simulink library "inp"  (R2021b)
settings: Solver=VariableStepAuto  StartTime=0.0  StopTime=10.0  RelTol=1e-3
undefined symbols (not defined in the file): C_TASK_5MS_S, FALSE, KINP_AcoreReadyToSlp_flg_ovrdflg, KINP_AcoreReadyToSlp_flg_ovrdval, KINP_AllowMovThd_OTA_enum_ovrdflg, KINP_AllowMovThd_OTA_enum_ovrdval, KINP_APSAngleTarget_Deg_ovrdflg, KINP_APSAngleTarget_Deg_ovrdval, KINP_APSDecReq_mps2_ovrdflg, KINP_APSDecReq_mps2_ovrdval, KINP_APSDecReqA_flg_ovrdflg, KINP_APSDecReqA_flg_ovrdval, KINP_APSDFLL_cm_ovrdflg, KINP_APSDFLL_cm_ovrdval, KINP_APSDFLR_cm_ovrdflg, KINP_APSDFLR_cm_ovrdval, KINP_APSDRLL_cm_ovrdflg, KINP_APSDRLL_cm_ovrdval, KINP_APSDRLR_cm_ovrdflg, KINP_APSDRLR_cm_ovrdval, KINP_APSExitCondition_enum_ovrdflg, KINP_APSExitCondition_enum_ovrdval, KINP_APSHWVer_enum_ovrdflg, KINP_APSHWVer_enum_ovrdval, KINP_APSProgressPCT_pct_ovrdflg, KINP_APSProgressPCT_pct_ovrdval, KINP_APSPwrReq_enum_ovrdflg, KINP_APSPwrReq_enum_ovrdval, KINP_APSReq_enum_ovrdflg, KINP_APSReq_enum_ovrdval, KINP_APSRQDisplay_enum_ovrdflg, KINP_APSRQDisplay_enum_ovrdval, KINP_APSRqEPASCtrl_flg_ovrdflg, KINP_APSRqEPASCtrl_flg_ovrdval, KINP_APSShiftPosnReq_enum_ovrdval, KINP_APSShiftPosnReq_enum_ovrflg, KINP_APSSpeedCMD_kph_ovrdval, KINP_APSSpeedCMD_kph_ovrflg, KINP_APSStaSystem_enum_ovrdflg, KINP_APSStaSystem_enum_ovrdval, KINP_APSSWVer_enum_ovrdflg, KINP_APSSWVer_enum_ovrdval, KINP_APSVMCReqA_flg_ovrdval, KINP_APSVMCReqA_flg_ovrflg, KINP_APSVRqEPASCtrl_flg_ovrdflg, KINP_APSVRqEPASCtrl_flg_ovrdval, KINP_AuxBattVolmV_mV_ovrdflg, KINP_AuxBattVolmV_mV_ovrdval, KINP_CAASSta_enum_ovrdflg, KINP_CAASSta_enum_ovrdval, KINP_CAASVMCReqA_flg_ovrdval, KINP_CAASVMCReqA_flg_ovrflg, KINP_CAN1BusOff_flg_ovrdflg, KINP_CAN1BusOff_flg_ovrdval, KINP_CAN2BusOff_flg_ovrdflg, KINP_CAN2BusOff_flg_ovrdval, KINP_CAN3BusOff_flg_ovrdflg, KINP_CAN3BusOff_flg_ovrdval, KINP_CAN4BusOff_flg_ovrdflg, KINP_CAN4BusOff_flg_ovrdval ... (+152)
libraries: FVT_lib x1035, hcu_lib x1
(part 4 of 33)

== system inp/INP/CAN1/CreateBus ==
  inp_CanValid_bus : Inport
  inp_Hal_bus : Inport  Port=2
  UnitConverter_{1..13,16,18..27,29,31..32,34..35,41,43..55,58..60,62,64..65,68..73,75,77,80,82,84..85,87,89,92,94,97..100,102..107,109..111,116..117,120,122,124,128,130..134} (89 alike) : DataTypeConversion  OutDataTypeStr=boolean
  UnitConverter_{40,42,66..67,76,81,88,93,96,101,108,118..119,121,123,125,127,129} (18 alike) : DataTypeConversion  OutDataTypeStr=single
  UnitConverter_{14..15,17,28,30,33,36..39,56..57,61,63,74,78..79,83,86,90..91,95,112..115,126} (27 alike) : DataTypeConversion  OutDataTypeStr=uint8
  bus_creator : BusCreator  Inputs=134
  bus_selector : BusSelector  OutputSignals=VINP_CANMsgValidABM1_flg,VINP_CANMsgValidEPB1_flg,VINP_CANMsgValidEPS1_flg,VINP_CANMsgValidESC1_flg,VINP_CANMsgValidESC5_flg,VINP_CANMsgValideBST1_flg
  bus_selector_1 : BusSelector  OutputSignals=VINP_ABM1CSErr_flg,VINP_ABM1RCErr_flg,VINP_ABMPassengerODSSta_flg,VINP_ABMRearPassengerCTRODSSta_flg,VINP_ABMRearPassengerLHODSSta_flg,VINP_ABMRearPassengerRHODSSta_flg,VINP_AirBagFailCmd_flg,VINP_ChecksumABM1_enum,VINP_CrashOutputSts_enum,VINP_DriverSeatBeltCmd_flg,VINP_LifeCountABM1_enum,VINP_PABSwitchCmd_flg,VINP_PsngrSeatBeltCmd_flg,VINP_RCenterSeatBeltCmd_flg,VINP_RDriverSeatBeltCmd_flg,VINP_RPsngrSeatBeltCmd_flg,VINP_TLHPsngrSeatBeltCmd_flg,VINP_TRHPsngrSeatBeltCmd_flg,VINP_EPB1CSErr_flg,VINP_EPB1RCErr_flg,VINP_DOASta_flg,VINP_EPB1RC_enum,VINP_EPBCarWashMode_flg,VINP_EPBErrSta_enum,VINP_EPBExtApplyAvail_flg,VINP_EPBExtReleaseAvail_flg,VINP_EPBSta_enum,VINP_EPS1CSErr_flg,VINP_EPS1RCErr_flg,VINP_DriIntend_enum,VINP_EPSAOIControl_enum,VINP_EPSRC_enum,VINP_EpasFailed_enum,VINP_SASAngle_Deg,VINP_SASCAL_flg,VINP_SASSpeed_degps,VINP_SASSpeedValid_flg,VINP_SASV_flg,VINP_ESC1CSErr_flg,VINP_ESC1RCErr_flg,VINP_ABSActive_flg,VINP_ABSFailed_flg,VINP_ABSWnlmpSta_flg,VINP_AVHActive_flg,VINP_AVHFailed_flg,VINP_AmberWnlmpSta_flg,VINP_BTCSActive_flg,VINP_EBDActive_flg,VINP_EBDFailed_flg,VINP_ESC1CS_enum,VINP_ESC1RC_enum,VINP_ESCActive_flg,VINP_ESCBeepReq_flg,VINP_ESCFailed_flg,VINP_ESCOFFStatus_enum,VINP_ESCOfflmpSta_flg,VINP_ESCWnlmpSta_enum,VINP_ESSActive_flg,VINP_FrPTCSActive_flg,VINP_FrntAxlTrqReqDrv_Nm,VINP_GRADE_Deg,VINP_HBBActive_flg,VINP_HBBFailed_flg,VINP_HDDActive_flg,VINP_HDDFailed_flg,VINP_HSAActive_flg,VINP_HSAFailed_flg,VINP_LFPulseCount_enum,VINP_LFPulseCountV_flg,VINP_LFRawWhlSpeed_kph,VINP_LFRawWhlSpeedV_flg,VINP_LFWhlRotDir_enum,VINP_LRPulseCount_enum,VINP_LRPulseCountV_flg,VINP_LRRawWhlSpeed_kph,VINP_LRRawWhlSpeedV_flg,VINP_LRWhlRotDir_enum,VINP_PBAActive_flg,VINP_PBAFailed_flg,VINP_RFPulseCount_enum,VINP_RFPulseCountV_flg,VINP_RFRawWhlSpeed_kph,VINP_RFRawWhlSpeedV_flg,VINP_RFWhlRotDir_enum,VINP_RRPulseCount_enum,VINP_RRPulseCountV_flg,VINP_RRRawWhlSpeed_kph,VINP_RRRawWhlSpeedV_flg,VINP_RRWhlRotDir_enum,VINP_RearAxlTrqReqDrv_Nm,VINP_RedWnlmpSta_flg,VINP_RrPTCSActive_flg,VINP_TCSActive_flg,VINP_TCSFailed_flg,VINP_VehSpeed_kph,VINP_ESC5CSErr_flg,VINP_ESC5RCErr_flg,VINP_ACCAvail_flg,VINP_AEBAvail_flg,VINP_ActBrkLampSta_flg,VINP_BrkDiscTempSta_flg,VINP_BrkPedalPos_pct,VINP_BrkPedalPosSta_flg,VINP_BrkSwSta_flg,VINP_BrkSwV_flg,VINP_ESC5CS_enum,VINP_ESC5RC_enum,VINP_ESCADASSta_enum,VINP_ESCAPSSta_enum,VINP_ESCStandstill_flg,VINP_FrRBCActive_flg,VINP_FrntAxlTrqReqBrk_Nm,VINP_LatAccel_Gps,VINP_LatAccelV_flg,VINP_LongAccel_Gps,VINP_LongAccelV_flg,VINP_MCPressure_bar,VINP_MCPressureV_flg,VINP_MeterIndVehSpeed_kph,VINP_RDCActive_enum,VINP_RearAxlTrqReqBrk_Nm,VINP_RrRBCActive_flg,VINP_YawRate_degps,VINP_YawRateV_flg,VINP_LowBrakeFluidSta_flg,VINP_eBSTAmberWnlmpSta_flg,VINP_eBSTBeepReq_flg,VINP_eBSTRedWnlmpSta_flg
  BINP_outputs : Outport
  wires:
  inp_CanValid_bus/1 -> [inp_CanValid_bus]
  inp_Hal_bus/1 -> [inp_Hal_bus]
  bus_selector/1 -> UnitConverter_1/1  "<VINP_CANMsgValidABM1_flg>"
  UnitConverter_1/1 -> bus_creator/1  "VINP_CANMsgValidABM1_flg"
  bus_selector/2 -> UnitConverter_2/1  "<VINP_CANMsgValidEPB1_flg>"
  UnitConverter_2/1 -> bus_creator/2  "VINP_CANMsgValidEPB1_flg"
  bus_selector/3 -> UnitConverter_3/1  "<VINP_CANMsgValidEPS1_flg>"
  UnitConverter_3/1 -> bus_creator/3  "VINP_CANMsgValidEPS1_flg"
  bus_selector/4 -> UnitConverter_4/1  "<VINP_CANMsgValidESC1_flg>"
  UnitConverter_4/1 -> bus_creator/4  "VINP_CANMsgValidESC1_flg"
  bus_selector/5 -> UnitConverter_5/1  "<VINP_CANMsgValidESC5_flg>"
  UnitConverter_5/1 -> bus_creator/5  "VINP_CANMsgValidESC5_flg"
  bus_selector/6 -> UnitConverter_6/1  "<VINP_CANMsgValideBST1_flg>"
  UnitConverter_6/1 -> bus_creator/6  "VINP_CANMsgValideBST1_flg"
  bus_selector_1/1 -> UnitConverter_7/1  "<VINP_ABM1CSErr_flg>"
  UnitConverter_7/1 -> bus_creator/7  "VINP_ABM1CSErr_flg"
  bus_selector_1/2 -> UnitConverter_8/1  "<VINP_ABM1RCErr_flg>"
  UnitConverter_8/1 -> bus_creator/8  "VINP_ABM1RCErr_flg"
  bus_selector_1/3 -> UnitConverter_9/1  "<VINP_ABMPassengerODSSta_flg>"
  UnitConverter_9/1 -> bus_creator/9  "VINP_ABMPassengerODSSta_flg"
  bus_selector_1/4 -> UnitConverter_10/1  "<VINP_ABMRearPassengerCTRODSSta_flg>"
  UnitConverter_10/1 -> bus_creator/10  "VINP_ABMRearPassengerCTRODSSta_flg"
  bus_selector_1/5 -> UnitConverter_11/1  "<VINP_ABMRearPassengerLHODSSta_flg>"
  UnitConverter_11/1 -> bus_creator/11  "VINP_ABMRearPassengerLHODSSta_flg"
  bus_selector_1/6 -> UnitConverter_12/1  "<VINP_ABMRearPassengerRHODSSta_flg>"
  UnitConverter_12/1 -> bus_creator/12  "VINP_ABMRearPassengerRHODSSta_flg"
  bus_selector_1/7 -> UnitConverter_13/1  "<VINP_AirBagFailCmd_flg>"
  UnitConverter_13/1 -> bus_creator/13  "VINP_AirBagFailCmd_flg"
  bus_selector_1/8 -> UnitConverter_14/1  "<VINP_ChecksumABM1_enum>"
  UnitConverter_14/1 -> bus_creator/14  "VINP_ChecksumABM1_enum"
  bus_selector_1/9 -> UnitConverter_15/1  "<VINP_CrashOutputSts_enum>"
  UnitConverter_15/1 -> bus_creator/15  "VINP_CrashOutputSts_enum"
  bus_selector_1/10 -> UnitConverter_16/1  "<VINP_DriverSeatBeltCmd_flg>"
  UnitConverter_16/1 -> bus_creator/16  "VINP_DriverSeatBeltCmd_flg"
  bus_selector_1/11 -> UnitConverter_17/1  "<VINP_LifeCountABM1_enum>"
  UnitConverter_17/1 -> bus_creator/17  "VINP_LifeCountABM1_enum"
  bus_selector_1/12 -> UnitConverter_18/1  "<VINP_PABSwitchCmd_flg>"
  UnitConverter_18/1 -> bus_creator/18  "VINP_PABSwitchCmd_flg"
  bus_selector_1/13 -> UnitConverter_19/1  "<VINP_PsngrSeatBeltCmd_flg>"
  UnitConverter_19/1 -> bus_creator/19  "VINP_PsngrSeatBeltCmd_flg"
  bus_selector_1/14 -> UnitConverter_20/1  "<VINP_RCenterSeatBeltCmd_flg>"
  UnitConverter_20/1 -> bus_creator/20  "VINP_RCenterSeatBeltCmd_flg"
  bus_selector_1/15 -> UnitConverter_21/1  "<VINP_RDriverSeatBeltCmd_flg>"
  UnitConverter_21/1 -> bus_creator/21  "VINP_RDriverSeatBeltCmd_flg"
  bus_selector_1/16 -> UnitConverter_22/1  "<VINP_RPsngrSeatBeltCmd_flg>"
  UnitConverter_22/1 -> bus_creator/22  "VINP_RPsngrSeatBeltCmd_flg"
  bus_selector_1/17 -> UnitConverter_23/1  "<VINP_TLHPsngrSeatBeltCmd_flg>"
  UnitConverter_23/1 -> bus_creator/23  "VINP_TLHPsngrSeatBeltCmd_flg"
  bus_selector_1/18 -> UnitConverter_24/1  "<VINP_TRHPsngrSeatBeltCmd_flg>"
  UnitConverter_24/1 -> bus_creator/24  "VINP_TRHPsngrSeatBeltCmd_flg"
  bus_selector_1/19 -> UnitConverter_25/1  "<VINP_EPB1CSErr_flg>"
  UnitConverter_25/1 -> bus_creator/25  "VINP_EPB1CSErr_flg"
  bus_selector_1/20 -> UnitConverter_26/1  "<VINP_EPB1RCErr_flg>"
  UnitConverter_26/1 -> bus_creator/26  "VINP_EPB1RCErr_flg"
  bus_selector_1/21 -> UnitConverter_27/1  "<VINP_DOASta_flg>"
  UnitConverter_27/1 -> bus_creator/27  "VINP_DOASta_flg"
  bus_selector_1/22 -> UnitConverter_28/1  "<VINP_EPB1RC_enum>"
  UnitConverter_28/1 -> bus_creator/28  "VINP_EPB1RC_enum"
  bus_selector_1/23 -> UnitConverter_29/1  "<VINP_EPBCarWashMode_flg>"
  UnitConverter_29/1 -> bus_creator/29  "VINP_EPBCarWashMode_flg"
  bus_selector_1/24 -> UnitConverter_30/1  "<VINP_EPBErrSta_enum>"
  UnitConverter_30/1 -> bus_creator/30  "VINP_EPBErrSta_enum"
  bus_selector_1/25 -> UnitConverter_31/1  "<VINP_EPBExtApplyAvail_flg>"
  UnitConverter_31/1 -> bus_creator/31  "VINP_EPBExtApplyAvail_flg"
  bus_selector_1/26 -> UnitConverter_32/1  "<VINP_EPBExtReleaseAvail_flg>"
  UnitConverter_32/1 -> bus_creator/32  "VINP_EPBExtReleaseAvail_flg"
  bus_selector_1/27 -> UnitConverter_33/1  "<VINP_EPBSta_enum>"
  UnitConverter_33/1 -> bus_creator/33  "VINP_EPBSta_enum"
  bus_selector_1/28 -> UnitConverter_34/1  "<VINP_EPS1CSErr_flg>"
  UnitConverter_34/1 -> bus_creator/34  "VINP_EPS1CSErr_flg"
  bus_selector_1/29 -> UnitConverter_35/1  "<VINP_EPS1RCErr_flg>"
  UnitConverter_35/1 -> bus_creator/35  "VINP_EPS1RCErr_flg"
  bus_selector_1/30 -> UnitConverter_36/1  "<VINP_DriIntend_enum>"
  UnitConverter_36/1 -> bus_creator/36  "VINP_DriIntend_enum"
  bus_selector_1/31 -> UnitConverter_37/1  "<VINP_EPSAOIControl_enum>"
  UnitConverter_37/1 -> bus_creator/37  "VINP_EPSAOIControl_enum"
  bus_selector_1/32 -> UnitConverter_38/1  "<VINP_EPSRC_enum>"
  UnitConverter_38/1 -> bus_creator/38  "VINP_EPSRC_enum"
  bus_selector_1/33 -> UnitConverter_39/1  "<VINP_EpasFailed_enum>"
  UnitConverter_39/1 -> bus_creator/39  "VINP_EpasFailed_enum"
  bus_selector_1/34 -> UnitConverter_40/1  "<VINP_SASAngle_Deg>"
  UnitConverter_40/1 -> bus_creator/40  "VINP_SASAngle_Deg"
  bus_selector_1/35 -> UnitConverter_41/1  "<VINP_SASCAL_flg>"
  UnitConverter_41/1 -> bus_creator/41  "VINP_SASCAL_flg"
  bus_selector_1/36 -> UnitConverter_42/1  "<VINP_SASSpeed_degps>"
  UnitConverter_42/1 -> bus_creator/42  "VINP_SASSpeed_degps"
  bus_selector_1/37 -> UnitConverter_43/1  "<VINP_SASSpeedValid_flg>"
  UnitConverter_43/1 -> bus_creator/43  "VINP_SASSpeedValid_flg"
  bus_selector_1/38 -> UnitConverter_44/1  "<VINP_SASV_flg>"
  UnitConverter_44/1 -> bus_creator/44  "VINP_SASV_flg"
  bus_selector_1/39 -> UnitConverter_45/1  "<VINP_ESC1CSErr_flg>"
  UnitConverter_45/1 -> bus_creator/45  "VINP_ESC1CSErr_flg"
  bus_selector_1/40 -> UnitConverter_46/1  "<VINP_ESC1RCErr_flg>"
  UnitConverter_46/1 -> bus_creator/46  "VINP_ESC1RCErr_flg"
  bus_selector_1/41 -> UnitConverter_47/1  "<VINP_ABSActive_flg>"
  UnitConverter_47/1 -> bus_creator/47  "VINP_ABSActive_flg"
  bus_selector_1/42 -> UnitConverter_48/1  "<VINP_ABSFailed_flg>"
  UnitConverter_48/1 -> bus_creator/48  "VINP_ABSFailed_flg"
  bus_selector_1/43 -> UnitConverter_49/1  "<VINP_ABSWnlmpSta_flg>"
  UnitConverter_49/1 -> bus_creator/49  "VINP_ABSWnlmpSta_flg"
  bus_selector_1/44 -> UnitConverter_50/1  "<VINP_AVHActive_flg>"
  UnitConverter_50/1 -> bus_creator/50  "VINP_AVHActive_flg"
  bus_selector_1/45 -> UnitConverter_51/1  "<VINP_AVHFailed_flg>"
  UnitConverter_51/1 -> bus_creator/51  "VINP_AVHFailed_flg"
  bus_selector_1/46 -> UnitConverter_52/1  "<VINP_AmberWnlmpSta_flg>"
  UnitConverter_52/1 -> bus_creator/52  "VINP_AmberWnlmpSta_flg"
  bus_selector_1/47 -> UnitConverter_53/1  "<VINP_BTCSActive_flg>"
  UnitConverter_53/1 -> bus_creator/53  "VINP_BTCSActive_flg"
  bus_selector_1/48 -> UnitConverter_54/1  "<VINP_EBDActive_flg>"
  UnitConverter_54/1 -> bus_creator/54  "VINP_EBDActive_flg"
  bus_selector_1/49 -> UnitConverter_55/1  "<VINP_EBDFailed_flg>"
  UnitConverter_55/1 -> bus_creator/55  "VINP_EBDFailed_flg"
  bus_selector_1/50 -> UnitConverter_56/1  "<VINP_ESC1CS_enum>"
  UnitConverter_56/1 -> bus_creator/56  "VINP_ESC1CS_enum"
  bus_selector_1/51 -> UnitConverter_57/1  "<VINP_ESC1RC_enum>"
  UnitConverter_57/1 -> bus_creator/57  "VINP_ESC1RC_enum"
  bus_selector_1/52 -> UnitConverter_58/1  "<VINP_ESCActive_flg>"
  UnitConverter_58/1 -> bus_creator/58  "VINP_ESCActive_flg"
  bus_selector_1/53 -> UnitConverter_59/1  "<VINP_ESCBeepReq_flg>"
  UnitConverter_59/1 -> bus_creator/59  "VINP_ESCBeepReq_flg"
  bus_selector_1/54 -> UnitConverter_60/1  "<VINP_ESCFailed_flg>"
  UnitConverter_60/1 -> bus_creator/60  "VINP_ESCFailed_flg"
  bus_selector_1/55 -> UnitConverter_61/1  "<VINP_ESCOFFStatus_enum>"
  UnitConverter_61/1 -> bus_creator/61  "VINP_ESCOFFStatus_enum"
  bus_selector_1/56 -> UnitConverter_62/1  "<VINP_ESCOfflmpSta_flg>"
  UnitConverter_62/1 -> bus_creator/62  "VINP_ESCOfflmpSta_flg"
  bus_selector_1/57 -> UnitConverter_63/1  "<VINP_ESCWnlmpSta_enum>"
  UnitConverter_63/1 -> bus_creator/63  "VINP_ESCWnlmpSta_enum"
  bus_selector_1/58 -> UnitConverter_64/1  "<VINP_ESSActive_flg>"
  UnitConverter_64/1 -> bus_creator/64  "VINP_ESSActive_flg"
  bus_selector_1/59 -> UnitConverter_65/1  "<VINP_FrPTCSActive_flg>"
  UnitConverter_65/1 -> bus_creator/65  "VINP_FrPTCSActive_flg"
  bus_selector_1/60 -> UnitConverter_66/1  "<VINP_FrntAxlTrqReqDrv_Nm>"
  UnitConverter_66/1 -> bus_creator/66  "VINP_FrntAxlTrqReqDrv_Nm"
  bus_selector_1/61 -> UnitConverter_67/1  "<VINP_GRADE_Deg>"
  UnitConverter_67/1 -> bus_creator/67  "VINP_GRADE_Deg"
  bus_selector_1/62 -> UnitConverter_68/1  "<VINP_HBBActive_flg>"
  UnitConverter_68/1 -> bus_creator/68  "VINP_HBBActive_flg"
  bus_selector_1/63 -> UnitConverter_69/1  "<VINP_HBBFailed_flg>"
  UnitConverter_69/1 -> bus_creator/69  "VINP_HBBFailed_flg"
  bus_selector_1/64 -> UnitConverter_70/1  "<VINP_HDDActive_flg>"
  UnitConverter_70/1 -> bus_creator/70  "VINP_HDDActive_flg"
  bus_selector_1/65 -> UnitConverter_71/1  "<VINP_HDDFailed_flg>"
  UnitConverter_71/1 -> bus_creator/71  "VINP_HDDFailed_flg"
  bus_selector_1/66 -> UnitConverter_72/1  "<VINP_HSAActive_flg>"
  UnitConverter_72/1 -> bus_creator/72  "VINP_HSAActive_flg"
  bus_selector_1/67 -> UnitConverter_73/1  "<VINP_HSAFailed_flg>"
  UnitConverter_73/1 -> bus_creator/73  "VINP_HSAFailed_flg"
  bus_selector_1/68 -> UnitConverter_74/1  "<VINP_LFPulseCount_enum>"
  UnitConverter_74/1 -> bus_creator/74  "VINP_LFPulseCount_enum"
  bus_selector_1/69 -> UnitConverter_75/1  "<VINP_LFPulseCountV_flg>"
  UnitConverter_75/1 -> bus_creator/75  "VINP_LFPulseCountV_flg"
  bus_selector_1/70 -> UnitConverter_76/1  "<VINP_LFRawWhlSpeed_kph>"
  UnitConverter_76/1 -> bus_creator/76  "VINP_LFRawWhlSpeed_kph"
  bus_selector_1/71 -> UnitConverter_77/1  "<VINP_LFRawWhlSpeedV_flg>"
  UnitConverter_77/1 -> bus_creator/77  "VINP_LFRawWhlSpeedV_flg"
  bus_selector_1/72 -> UnitConverter_78/1  "<VINP_LFWhlRotDir_enum>"
  UnitConverter_78/1 -> bus_creator/78  "VINP_LFWhlRotDir_enum"
  bus_selector_1/73 -> UnitConverter_79/1  "<VINP_LRPulseCount_enum>"
  UnitConverter_79/1 -> bus_creator/79  "VINP_LRPulseCount_enum"
  bus_selector_1/74 -> UnitConverter_80/1  "<VINP_LRPulseCountV_flg>"
  UnitConverter_80/1 -> bus_creator/80  "VINP_LRPulseCountV_flg"
  bus_selector_1/75 -> UnitConverter_81/1  "<VINP_LRRawWhlSpeed_kph>"
  UnitConverter_81/1 -> bus_creator/81  "VINP_LRRawWhlSpeed_kph"
  bus_selector_1/76 -> UnitConverter_82/1  "<VINP_LRRawWhlSpeedV_flg>"
  UnitConverter_82/1 -> bus_creator/82  "VINP_LRRawWhlSpeedV_flg"
  bus_selector_1/77 -> UnitConverter_83/1  "<VINP_LRWhlRotDir_enum>"
  UnitConverter_83/1 -> bus_creator/83  "VINP_LRWhlRotDir_enum"
  bus_selector_1/78 -> UnitConverter_84/1  "<VINP_PBAActive_flg>"
  UnitConverter_84/1 -> bus_creator/84  "VINP_PBAActive_flg"
  bus_selector_1/79 -> UnitConverter_85/1  "<VINP_PBAFailed_flg>"
  UnitConverter_85/1 -> bus_creator/85  "VINP_PBAFailed_flg"
  bus_selector_1/80 -> UnitConverter_86/1  "<VINP_RFPulseCount_enum>"
  UnitConverter_86/1 -> bus_creator/86  "VINP_RFPulseCount_enum"
  bus_selector_1/81 -> UnitConverter_87/1  "<VINP_RFPulseCountV_flg>"
  UnitConverter_87/1 -> bus_creator/87  "VINP_RFPulseCountV_flg"
  bus_selector_1/82 -> UnitConverter_88/1  "<VINP_RFRawWhlSpeed_kph>"
  UnitConverter_88/1 -> bus_creator/88  "VINP_RFRawWhlSpeed_kph"
  bus_selector_1/83 -> UnitConverter_89/1  "<VINP_RFRawWhlSpeedV_flg>"
  UnitConverter_89/1 -> bus_creator/89  "VINP_RFRawWhlSpeedV_flg"
  bus_selector_1/84 -> UnitConverter_90/1  "<VINP_RFWhlRotDir_enum>"
  UnitConverter_90/1 -> bus_creator/90  "VINP_RFWhlRotDir_enum"
  bus_selector_1/85 -> UnitConverter_91/1  "<VINP_RRPulseCount_enum>"
  UnitConverter_91/1 -> bus_creator/91  "VINP_RRPulseCount_enum"
  bus_selector_1/86 -> UnitConverter_92/1  "<VINP_RRPulseCountV_flg>"
  UnitConverter_92/1 -> bus_creator/92  "VINP_RRPulseCountV_flg"
  bus_selector_1/87 -> UnitConverter_93/1  "<VINP_RRRawWhlSpeed_kph>"
  UnitConverter_93/1 -> bus_creator/93  "VINP_RRRawWhlSpeed_kph"
  bus_selector_1/88 -> UnitConverter_94/1  "<VINP_RRRawWhlSpeedV_flg>"
  UnitConverter_94/1 -> bus_creator/94  "VINP_RRRawWhlSpeedV_flg"
  bus_selector_1/89 -> UnitConverter_95/1  "<VINP_RRWhlRotDir_enum>"
  UnitConverter_95/1 -> bus_creator/95  "VINP_RRWhlRotDir_enum"
  bus_selector_1/90 -> UnitConverter_96/1  "<VINP_RearAxlTrqReqDrv_Nm>"
  UnitConverter_96/1 -> bus_creator/96  "VINP_RearAxlTrqReqDrv_Nm"
  bus_selector_1/91 -> UnitConverter_97/1  "<VINP_RedWnlmpSta_flg>"
  UnitConverter_97/1 -> bus_creator/97  "VINP_RedWnlmpSta_flg"
  bus_selector_1/92 -> UnitConverter_98/1  "<VINP_RrPTCSActive_flg>"
  UnitConverter_98/1 -> bus_creator/98  "VINP_RrPTCSActive_flg"
  bus_selector_1/93 -> UnitConverter_99/1  "<VINP_TCSActive_flg>"
  UnitConverter_99/1 -> bus_creator/99  "VINP_TCSActive_flg"
  bus_selector_1/94 -> UnitConverter_100/1  "<VINP_TCSFailed_flg>"
  UnitConverter_100/1 -> bus_creator/100  "VINP_TCSFailed_flg"
  bus_selector_1/95 -> UnitConverter_101/1  "<VINP_VehSpeed_kph>"
  UnitConverter_101/1 -> bus_creator/101  "VINP_VehSpeed_kph"
  bus_selector_1/96 -> UnitConverter_102/1  "<VINP_ESC5CSErr_flg>"
  UnitConverter_102/1 -> bus_creator/102  "VINP_ESC5CSErr_flg"
  bus_selector_1/97 -> UnitConverter_103/1  "<VINP_ESC5RCErr_flg>"
  UnitConverter_103/1 -> bus_creator/103  "VINP_ESC5RCErr_flg"
  bus_selector_1/98 -> UnitConverter_104/1  "<VINP_ACCAvail_flg>"
  UnitConverter_104/1 -> bus_creator/104  "VINP_ACCAvail_flg"
  bus_selector_1/99 -> UnitConverter_105/1  "<VINP_AEBAvail_flg>"
  UnitConverter_105/1 -> bus_creator/105  "VINP_AEBAvail_flg"
  bus_selector_1/100 -> UnitConverter_106/1  "<VINP_ActBrkLampSta_flg>"
  UnitConverter_106/1 -> bus_creator/106  "VINP_ActBrkLampSta_flg"
  bus_selector_1/101 -> UnitConverter_107/1  "<VINP_BrkDiscTempSta_flg>"
  UnitConverter_107/1 -> bus_creator/107  "VINP_BrkDiscTempSta_flg"
  bus_selector_1/102 -> UnitConverter_108/1  "<VINP_BrkPedalPos_pct>"
  UnitConverter_108/1 -> bus_creator/108  "VINP_BrkPedalPos_pct"
  bus_selector_1/103 -> UnitConverter_109/1  "<VINP_BrkPedalPosSta_flg>"
  UnitConverter_109/1 -> bus_creator/109  "VINP_BrkPedalPosSta_flg"
  bus_selector_1/104 -> UnitConverter_110/1  "<VINP_BrkSwSta_flg>"
  UnitConverter_110/1 -> bus_creator/110  "VINP_BrkSwSta_flg"
  bus_selector_1/105 -> UnitConverter_111/1  "<VINP_BrkSwV_flg>"
  UnitConverter_111/1 -> bus_creator/111  "VINP_BrkSwV_flg"
  bus_selector_1/106 -> UnitConverter_112/1  "<VINP_ESC5CS_enum>"
  UnitConverter_112/1 -> bus_creator/112  "VINP_ESC5CS_enum"
  bus_selector_1/107 -> UnitConverter_113/1  "<VINP_ESC5RC_enum>"
  UnitConverter_113/1 -> bus_creator/113  "VINP_ESC5RC_enum"
  bus_selector_1/108 -> UnitConverter_114/1  "<VINP_ESCADASSta_enum>"
  UnitConverter_114/1 -> bus_creator/114  "VINP_ESCADASSta_enum"
  bus_selector_1/109 -> UnitConverter_115/1  "<VINP_ESCAPSSta_enum>"
  UnitConverter_115/1 -> bus_creator/115  "VINP_ESCAPSSta_enum"
  bus_selector_1/110 -> UnitConverter_116/1  "<VINP_ESCStandstill_flg>"
  UnitConverter_116/1 -> bus_creator/116  "VINP_ESCStandstill_flg"
  bus_selector_1/111 -> UnitConverter_117/1  "<VINP_FrRBCActive_flg>"
  UnitConverter_117/1 -> bus_creator/117  "VINP_FrRBCActive_flg"
  bus_selector_1/112 -> UnitConverter_118/1  "<VINP_FrntAxlTrqReqBrk_Nm>"
  UnitConverter_118/1 -> bus_creator/118  "VINP_FrntAxlTrqReqBrk_Nm"
  bus_selector_1/113 -> UnitConverter_119/1  "<VINP_LatAccel_Gps>"
  UnitConverter_119/1 -> bus_creator/119  "VINP_LatAccel_Gps"
  bus_selector_1/114 -> UnitConverter_120/1  "<VINP_LatAccelV_flg>"
  UnitConverter_120/1 -> bus_creator/120  "VINP_LatAccelV_flg"
  bus_selector_1/115 -> UnitConverter_121/1  "<VINP_LongAccel_Gps>"
  UnitConverter_121/1 -> bus_creator/121  "VINP_LongAccel_Gps"
  bus_selector_1/116 -> UnitConverter_122/1  "<VINP_LongAccelV_flg>"
  UnitConverter_122/1 -> bus_creator/122  "VINP_LongAccelV_flg"
  bus_selector_1/117 -> UnitConverter_123/1  "<VINP_MCPressure_bar>"
  UnitConverter_123/1 -> bus_creator/123  "VINP_MCPressure_bar"
  bus_selector_1/118 -> UnitConverter_124/1  "<VINP_MCPressureV_flg>"
  UnitConverter_124/1 -> bus_creator/124  "VINP_MCPressureV_flg"
  bus_selector_1/119 -> UnitConverter_125/1  "<VINP_MeterIndVehSpeed_kph>"
  UnitConverter_125/1 -> bus_creator/125  "VINP_MeterIndVehSpeed_kph"
  bus_selector_1/120 -> UnitConverter_126/1  "<VINP_RDCActive_enum>"
  UnitConverter_126/1 -> bus_creator/126  "VINP_RDCActive_enum"
  bus_selector_1/121 -> UnitConverter_127/1  "<VINP_RearAxlTrqReqBrk_Nm>"
  UnitConverter_127/1 -> bus_creator/127  "VINP_RearAxlTrqReqBrk_Nm"
  bus_selector_1/122 -> UnitConverter_128/1  "<VINP_RrRBCActive_flg>"
  UnitConverter_128/1 -> bus_creator/128  "VINP_RrRBCActive_flg"
  bus_selector_1/123 -> UnitConverter_129/1  "<VINP_YawRate_degps>"
  UnitConverter_129/1 -> bus_creator/129  "VINP_YawRate_degps"
  bus_selector_1/124 -> UnitConverter_130/1  "<VINP_YawRateV_flg>"
  UnitConverter_130/1 -> bus_creator/130  "VINP_YawRateV_flg"
  bus_selector_1/125 -> UnitConverter_131/1  "<VINP_LowBrakeFluidSta_flg>"
  UnitConverter_131/1 -> bus_creator/131  "VINP_LowBrakeFluidSta_flg"
  bus_selector_1/126 -> UnitConverter_132/1  "<VINP_eBSTAmberWnlmpSta_flg>"
  UnitConverter_132/1 -> bus_creator/132  "VINP_eBSTAmberWnlmpSta_flg"
  bus_selector_1/127 -> UnitConverter_133/1  "<VINP_eBSTBeepReq_flg>"
  UnitConverter_133/1 -> bus_creator/133  "VINP_eBSTBeepReq_flg"
  bus_selector_1/128 -> UnitConverter_134/1  "<VINP_eBSTRedWnlmpSta_flg>"
  UnitConverter_134/1 -> bus_creator/134  "VINP_eBSTRedWnlmpSta_flg"
  [inp_CanValid_bus] -> bus_selector/1
  [inp_Hal_bus] -> bus_selector_1/1
  bus_creator/1 -> BINP_outputs/1

== system inp/INP/CAN1/SignalCheck ==
  inp_CanValid_bus : Inport
  TASK_TIME_S : Inport  Port=2
  BHAL_outputs : Inport  Port=3
  ABM1 : Subsystem
  EPB1 : Subsystem
  EPS1 : Subsystem
  ESC1 : Subsystem
  ESC5 : Subsystem
  bus_creator : BusCreator  Inputs=128
  eBST1 : Subsystem
  inp_Hal_bus : Outport
  wires:
  inp_CanValid_bus/1 -> [inp_CanValid_bus]
  TASK_TIME_S/1 -> [TASK_TIME_S]
  BHAL_outputs/1 -> [BHAL_outputs]
  [BHAL_outputs] -> ABM1/1(BHAL_outputs)
  [inp_CanValid_bus] -> ABM1/2(inp_CanValid_bus)
  ABM1/1(VINP_ABM1CSErr_flg) -> [VINP_ABM1CSErr_flg]
  ABM1/2(VINP_ABM1RCErr_flg) -> [VINP_ABM1RCErr_flg]
  ABM1/3(VINP_ABMPassengerODSSta_flg) -> [VINP_ABMPassengerODSSta_flg]
  ABM1/4(VINP_ABMRearPassengerCTRODSSta_flg) -> [VINP_ABMRearPassengerCTRODSSta_flg]
  ABM1/5(VINP_ABMRearPassengerLHODSSta_flg) -> [VINP_ABMRearPassengerLHODSSta_flg]
  ABM1/6(VINP_ABMRearPassengerRHODSSta_flg) -> [VINP_ABMRearPassengerRHODSSta_flg]
  ABM1/7(VINP_AirBagFailCmd_flg) -> [VINP_AirBagFailCmd_flg]
  ABM1/8(VINP_ChecksumABM1_enum) -> [VINP_ChecksumABM1_enum]
  ABM1/9(VINP_CrashOutputSts_enum) -> [VINP_CrashOutputSts_enum]
  ABM1/10(VINP_DriverSeatBeltCmd_flg) -> [VINP_DriverSeatBeltCmd_flg]
  ABM1/11(VINP_LifeCountABM1_enum) -> [VINP_LifeCountABM1_enum]
  ABM1/12(VINP_PABSwitchCmd_flg) -> [VINP_PABSwitchCmd_flg]
  ABM1/13(VINP_PsngrSeatBeltCmd_flg) -> [VINP_PsngrSeatBeltCmd_flg]
  ABM1/14(VINP_RCenterSeatBeltCmd_flg) -> [VINP_RCenterSeatBeltCmd_flg]
  ABM1/15(VINP_RDriverSeatBeltCmd_flg) -> [VINP_RDriverSeatBeltCmd_flg]
  ABM1/16(VINP_RPsngrSeatBeltCmd_flg) -> [VINP_RPsngrSeatBeltCmd_flg]
  ABM1/17(VINP_TLHPsngrSeatBeltCmd_flg) -> [VINP_TLHPsngrSeatBeltCmd_flg]
  ABM1/18(VINP_TRHPsngrSeatBeltCmd_flg) -> [VINP_TRHPsngrSeatBeltCmd_flg]
  [BHAL_outputs] -> EPB1/1(BHAL_outputs)
  [inp_CanValid_bus] -> EPB1/2(inp_CanValid_bus)
  EPB1/1(VINP_EPB1CSErr_flg) -> [VINP_EPB1CSErr_flg]
  EPB1/2(VINP_EPB1RCErr_flg) -> [VINP_EPB1RCErr_flg]
  EPB1/3(VINP_DOASta_flg) -> [VINP_DOASta_flg]
  EPB1/4(VINP_EPB1RC_enum) -> [VINP_EPB1RC_enum]
  EPB1/5(VINP_EPBCarWashMode_flg) -> [VINP_EPBCarWashMode_flg]
  EPB1/6(VINP_EPBErrSta_enum) -> [VINP_EPBErrSta_enum]
  EPB1/7(VINP_EPBExtApplyAvail_flg) -> [VINP_EPBExtApplyAvail_flg]
  EPB1/8(VINP_EPBExtReleaseAvail_flg) -> [VINP_EPBExtReleaseAvail_flg]
  EPB1/9(VINP_EPBSta_enum) -> [VINP_EPBSta_enum]
  [BHAL_outputs] -> EPS1/1(BHAL_outputs)
  [inp_CanValid_bus] -> EPS1/2(inp_CanValid_bus)
  EPS1/1(VINP_EPS1CSErr_flg) -> [VINP_EPS1CSErr_flg]
  EPS1/2(VINP_EPS1RCErr_flg) -> [VINP_EPS1RCErr_flg]
  EPS1/3(VINP_DriIntend_enum) -> [VINP_DriIntend_enum]
  EPS1/4(VINP_EPSAOIControl_enum) -> [VINP_EPSAOIControl_enum]
  EPS1/5(VINP_EPSRC_enum) -> [VINP_EPSRC_enum]
  EPS1/6(VINP_EpasFailed_enum) -> [VINP_EpasFailed_enum]
  EPS1/7(VINP_SASAngle_Deg) -> [VINP_SASAngle_Deg]
  EPS1/8(VINP_SASCAL_flg) -> [VINP_SASCAL_flg]
  EPS1/9(VINP_SASSpeed_degps) -> [VINP_SASSpeed_degps]
  EPS1/10(VINP_SASSpeedValid_flg) -> [VINP_SASSpeedValid_flg]
  EPS1/11(VINP_SASV_flg) -> [VINP_SASV_flg]
  [BHAL_outputs] -> ESC1/1(BHAL_outputs)
  [inp_CanValid_bus] -> ESC1/2(inp_CanValid_bus)
  ESC1/1(VINP_ESC1CSErr_flg) -> [VINP_ESC1CSErr_flg]
  ESC1/2(VINP_ESC1RCErr_flg) -> [VINP_ESC1RCErr_flg]
  ESC1/3(VINP_ABSActive_flg) -> [VINP_ABSActive_flg]
  ESC1/4(VINP_ABSFailed_flg) -> [VINP_ABSFailed_flg]
  ESC1/5(VINP_ABSWnlmpSta_flg) -> [VINP_ABSWnlmpSta_flg]
  ESC1/6(VINP_AVHActive_flg) -> [VINP_AVHActive_flg]
  ESC1/7(VINP_AVHFailed_flg) -> [VINP_AVHFailed_flg]
  ESC1/8(VINP_AmberWnlmpSta_flg) -> [VINP_AmberWnlmpSta_flg]
  ESC1/9(VINP_BTCSActive_flg) -> [VINP_BTCSActive_flg]
  ESC1/10(VINP_EBDActive_flg) -> [VINP_EBDActive_flg]
  ESC1/11(VINP_EBDFailed_flg) -> [VINP_EBDFailed_flg]
  ESC1/12(VINP_ESC1CS_enum) -> [VINP_ESC1CS_enum]
  ESC1/13(VINP_ESC1RC_enum) -> [VINP_ESC1RC_enum]
  ESC1/14(VINP_ESCActive_flg) -> [VINP_ESCActive_flg]
  ESC1/15(VINP_ESCBeepReq_flg) -> [VINP_ESCBeepReq_flg]
  ESC1/16(VINP_ESCFailed_flg) -> [VINP_ESCFailed_flg]
  ESC1/17(VINP_ESCOFFStatus_enum) -> [VINP_ESCOFFStatus_enum]
  ESC1/18(VINP_ESCOfflmpSta_flg) -> [VINP_ESCOfflmpSta_flg]
  ESC1/19(VINP_ESCWnlmpSta_enum) -> [VINP_ESCWnlmpSta_enum]
  ESC1/20(VINP_ESSActive_flg) -> [VINP_ESSActive_flg]
  ESC1/21(VINP_FrPTCSActive_flg) -> [VINP_FrPTCSActive_flg]
  ESC1/22(VINP_FrntAxlTrqReqDrv_Nm) -> [VINP_FrntAxlTrqReqDrv_Nm]
  ESC1/23(VINP_GRADE_Deg) -> [VINP_GRADE_Deg]
  ESC1/24(VINP_HBBActive_flg) -> [VINP_HBBActive_flg]
  ESC1/25(VINP_HBBFailed_flg) -> [VINP_HBBFailed_flg]
  ESC1/26(VINP_HDDActive_flg) -> [VINP_HDDActive_flg]
  ESC1/27(VINP_HDDFailed_flg) -> [VINP_HDDFailed_flg]
  ESC1/28(VINP_HSAActive_flg) -> [VINP_HSAActive_flg]
  ESC1/29(VINP_HSAFailed_flg) -> [VINP_HSAFailed_flg]
  ESC1/30(VINP_LFPulseCount_enum) -> [VINP_LFPulseCount_enum]
  ESC1/31(VINP_LFPulseCountV_flg) -> [VINP_LFPulseCountV_flg]
  ESC1/32(VINP_LFRawWhlSpeed_kph) -> [VINP_LFRawWhlSpeed_kph]
  ESC1/33(VINP_LFRawWhlSpeedV_flg) -> [VINP_LFRawWhlSpeedV_flg]
  ESC1/34(VINP_LFWhlRotDir_enum) -> [VINP_LFWhlRotDir_enum]
  ESC1/35(VINP_LRPulseCount_enum) -> [VINP_LRPulseCount_enum]
  ESC1/36(VINP_LRPulseCountV_flg) -> [VINP_LRPulseCountV_flg]
  ESC1/37(VINP_LRRawWhlSpeed_kph) -> [VINP_LRRawWhlSpeed_kph]
  ESC1/38(VINP_LRRawWhlSpeedV_flg) -> [VINP_LRRawWhlSpeedV_flg]
  ESC1/39(VINP_LRWhlRotDir_enum) -> [VINP_LRWhlRotDir_enum]
  ESC1/40(VINP_PBAActive_flg) -> [VINP_PBAActive_flg]
  ESC1/41(VINP_PBAFailed_flg) -> [VINP_PBAFailed_flg]
  ESC1/42(VINP_RFPulseCount_enum) -> [VINP_RFPulseCount_enum]
  ESC1/43(VINP_RFPulseCountV_flg) -> [VINP_RFPulseCountV_flg]
  ESC1/44(VINP_RFRawWhlSpeed_kph) -> [VINP_RFRawWhlSpeed_kph]
  ESC1/45(VINP_RFRawWhlSpeedV_flg) -> [VINP_RFRawWhlSpeedV_flg]
  ESC1/46(VINP_RFWhlRotDir_enum) -> [VINP_RFWhlRotDir_enum]
  ESC1/47(VINP_RRPulseCount_enum) -> [VINP_RRPulseCount_enum]
  ESC1/48(VINP_RRPulseCountV_flg) -> [VINP_RRPulseCountV_flg]
  ESC1/49(VINP_RRRawWhlSpeed_kph) -> [VINP_RRRawWhlSpeed_kph]
  ESC1/50(VINP_RRRawWhlSpeedV_flg) -> [VINP_RRRawWhlSpeedV_flg]
  ESC1/51(VINP_RRWhlRotDir_enum) -> [VINP_RRWhlRotDir_enum]
  ESC1/52(VINP_RearAxlTrqReqDrv_Nm) -> [VINP_RearAxlTrqReqDrv_Nm]
  ESC1/53(VINP_RedWnlmpSta_flg) -> [VINP_RedWnlmpSta_flg]
  ESC1/54(VINP_RrPTCSActive_flg) -> [VINP_RrPTCSActive_flg]
  ESC1/55(VINP_TCSActive_flg) -> [VINP_TCSActive_flg]
  ESC1/56(VINP_TCSFailed_flg) -> [VINP_TCSFailed_flg]
  ESC1/57(VINP_VehSpeed_kph) -> [VINP_VehSpeed_kph]
  [BHAL_outputs] -> ESC5/1(BHAL_outputs)
  [inp_CanValid_bus] -> ESC5/2(inp_CanValid_bus)
  ESC5/1(VINP_ESC5CSErr_flg) -> [VINP_ESC5CSErr_flg]
  ESC5/2(VINP_ESC5RCErr_flg) -> [VINP_ESC5RCErr_flg]
  ESC5/3(VINP_ACCAvail_flg) -> [VINP_ACCAvail_flg]
  ESC5/4(VINP_AEBAvail_flg) -> [VINP_AEBAvail_flg]
  ESC5/5(VINP_ActBrkLampSta_flg) -> [VINP_ActBrkLampSta_flg]
  ESC5/6(VINP_BrkDiscTempSta_flg) -> [VINP_BrkDiscTempSta_flg]
  ESC5/7(VINP_BrkPedalPos_pct) -> [VINP_BrkPedalPos_pct]
  ESC5/8(VINP_BrkPedalPosSta_flg) -> [VINP_BrkPedalPosSta_flg]
  ESC5/9(VINP_BrkSwSta_flg) -> [VINP_BrkSwSta_flg]
  ESC5/10(VINP_BrkSwV_flg) -> [VINP_BrkSwV_flg]
  ESC5/11(VINP_ESC5CS_enum) -> [VINP_ESC5CS_enum]
  ESC5/12(VINP_ESC5RC_enum) -> [VINP_ESC5RC_enum]
  ESC5/13(VINP_ESCADASSta_enum) -> [VINP_ESCADASSta_enum]
  ESC5/14(VINP_ESCAPSSta_enum) -> [VINP_ESCAPSSta_enum]
  ESC5/15(VINP_ESCStandstill_flg) -> [VINP_ESCStandstill_flg]
  ESC5/16(VINP_FrRBCActive_flg) -> [VINP_FrRBCActive_flg]
  ESC5/17(VINP_FrntAxlTrqReqBrk_Nm) -> [VINP_FrntAxlTrqReqBrk_Nm]
  ESC5/18(VINP_LatAccel_Gps) -> [VINP_LatAccel_Gps]
  ESC5/19(VINP_LatAccelV_flg) -> [VINP_LatAccelV_flg]
  ESC5/20(VINP_LongAccel_Gps) -> [VINP_LongAccel_Gps]
  ESC5/21(VINP_LongAccelV_flg) -> [VINP_LongAccelV_flg]
  ESC5/22(VINP_MCPressure_bar) -> [VINP_MCPressure_bar]
  ESC5/23(VINP_MCPressureV_flg) -> [VINP_MCPressureV_flg]
  ESC5/24(VINP_MeterIndVehSpeed_kph) -> [VINP_MeterIndVehSpeed_kph]
  ESC5/25(VINP_RDCActive_enum) -> [VINP_RDCActive_enum]
  ESC5/26(VINP_RearAxlTrqReqBrk_Nm) -> [VINP_RearAxlTrqReqBrk_Nm]
  ESC5/27(VINP_RrRBCActive_flg) -> [VINP_RrRBCActive_flg]
  ESC5/28(VINP_YawRate_degps) -> [VINP_YawRate_degps]
  ESC5/29(VINP_YawRateV_flg) -> [VINP_YawRateV_flg]
  [BHAL_outputs] -> eBST1/1(BHAL_outputs)
  [inp_CanValid_bus] -> eBST1/2(inp_CanValid_bus)
  eBST1/1(VINP_LowBrakeFluidSta_flg) -> [VINP_LowBrakeFluidSta_flg]
  eBST1/2(VINP_eBSTAmberWnlmpSta_flg) -> [VINP_eBSTAmberWnlmpSta_flg]
  eBST1/3(VINP_eBSTBeepReq_flg) -> [VINP_eBSTBeepReq_flg]
  eBST1/4(VINP_eBSTRedWnlmpSta_flg) -> [VINP_eBSTRedWnlmpSta_flg]
  bus_creator/1 -> inp_Hal_bus/1
  [VINP_ABM1CSErr_flg] -> bus_creator/1
  [VINP_ABM1RCErr_flg] -> bus_creator/2
  [VINP_ABMPassengerODSSta_flg] -> bus_creator/3
  [VINP_ABMRearPassengerCTRODSSta_flg] -> bus_creator/4
  [VINP_ABMRearPassengerLHODSSta_flg] -> bus_creator/5
  [VINP_ABMRearPassengerRHODSSta_flg] -> bus_creator/6
  [VINP_AirBagFailCmd_flg] -> bus_creator/7
  [VINP_ChecksumABM1_enum] -> bus_creator/8
  [VINP_CrashOutputSts_enum] -> bus_creator/9
  [VINP_DriverSeatBeltCmd_flg] -> bus_creator/10
  [VINP_LifeCountABM1_enum] -> bus_creator/11
  [VINP_PABSwitchCmd_flg] -> bus_creator/12
  [VINP_PsngrSeatBeltCmd_flg] -> bus_creator/13
  [VINP_RCenterSeatBeltCmd_flg] -> bus_creator/14
  [VINP_RDriverSeatBeltCmd_flg] -> bus_creator/15
  [VINP_RPsngrSeatBeltCmd_flg] -> bus_creator/16
  [VINP_TLHPsngrSeatBeltCmd_flg] -> bus_creator/17
  [VINP_TRHPsngrSeatBeltCmd_flg] -> bus_creator/18
  [VINP_EPB1CSErr_flg] -> bus_creator/19
  [VINP_EPB1RCErr_flg] -> bus_creator/20
  [VINP_DOASta_flg] -> bus_creator/21
  [VINP_EPB1RC_enum] -> bus_creator/22
  [VINP_EPBCarWashMode_flg] -> bus_creator/23
  [VINP_EPBErrSta_enum] -> bus_creator/24
  [VINP_EPBExtApplyAvail_flg] -> bus_creator/25
  [VINP_EPBExtReleaseAvail_flg] -> bus_creator/26
  [VINP_EPBSta_enum] -> bus_creator/27
  [VINP_EPS1CSErr_flg] -> bus_creator/28
  [VINP_EPS1RCErr_flg] -> bus_creator/29
  [VINP_DriIntend_enum] -> bus_creator/30
  [VINP_EPSAOIControl_enum] -> bus_creator/31
  [VINP_EPSRC_enum] -> bus_creator/32
  [VINP_EpasFailed_enum] -> bus_creator/33
  [VINP_SASAngle_Deg] -> bus_creator/34
  [VINP_SASCAL_flg] -> bus_creator/35
  [VINP_SASSpeed_degps] -> bus_creator/36
  [VINP_SASSpeedValid_flg] -> bus_creator/37
  [VINP_SASV_flg] -> bus_creator/38
  [VINP_ESC1CSErr_flg] -> bus_creator/39
  [VINP_ESC1RCErr_flg] -> bus_creator/40
  [VINP_ABSActive_flg] -> bus_creator/41
  [VINP_ABSFailed_flg] -> bus_creator/42
  [VINP_ABSWnlmpSta_flg] -> bus_creator/43
  [VINP_AVHActive_flg] -> bus_creator/44
  [VINP_AVHFailed_flg] -> bus_creator/45
  [VINP_AmberWnlmpSta_flg] -> bus_creator/46
  [VINP_BTCSActive_flg] -> bus_creator/47
  [VINP_EBDActive_flg] -> bus_creator/48
  [VINP_EBDFailed_flg] -> bus_creator/49
  [VINP_ESC1CS_enum] -> bus_creator/50
  [VINP_ESC1RC_enum] -> bus_creator/51
  [VINP_ESCActive_flg] -> bus_creator/52
  [VINP_ESCBeepReq_flg] -> bus_creator/53
  [VINP_ESCFailed_flg] -> bus_creator/54
  [VINP_ESCOFFStatus_enum] -> bus_creator/55
  [VINP_ESCOfflmpSta_flg] -> bus_creator/56
  [VINP_ESCWnlmpSta_enum] -> bus_creator/57
  [VINP_ESSActive_flg] -> bus_creator/58
  [VINP_FrPTCSActive_flg] -> bus_creator/59
  [VINP_FrntAxlTrqReqDrv_Nm] -> bus_creator/60
  [VINP_GRADE_Deg] -> bus_creator/61
  [VINP_HBBActive_flg] -> bus_creator/62
  [VINP_HBBFailed_flg] -> bus_creator/63
  [VINP_HDDActive_flg] -> bus_creator/64
  [VINP_HDDFailed_flg] -> bus_creator/65
  [VINP_HSAActive_flg] -> bus_creator/66
  [VINP_HSAFailed_flg] -> bus_creator/67
  [VINP_LFPulseCount_enum] -> bus_creator/68
  [VINP_LFPulseCountV_flg] -> bus_creator/69
  [VINP_LFRawWhlSpeed_kph] -> bus_creator/70
  [VINP_LFRawWhlSpeedV_flg] -> bus_creator/71
  [VINP_LFWhlRotDir_enum] -> bus_creator/72
  [VINP_LRPulseCount_enum] -> bus_creator/73
  [VINP_LRPulseCountV_flg] -> bus_creator/74
  [VINP_LRRawWhlSpeed_kph] -> bus_creator/75
  [VINP_LRRawWhlSpeedV_flg] -> bus_creator/76
  [VINP_LRWhlRotDir_enum] -> bus_creator/77
  [VINP_PBAActive_flg] -> bus_creator/78
  [VINP_PBAFailed_flg] -> bus_creator/79
  [VINP_RFPulseCount_enum] -> bus_creator/80
  [VINP_RFPulseCountV_flg] -> bus_creator/81
  [VINP_RFRawWhlSpeed_kph] -> bus_creator/82
  [VINP_RFRawWhlSpeedV_flg] -> bus_creator/83
  [VINP_RFWhlRotDir_enum] -> bus_creator/84
  [VINP_RRPulseCount_enum] -> bus_creator/85
  [VINP_RRPulseCountV_flg] -> bus_creator/86
  [VINP_RRRawWhlSpeed_kph] -> bus_creator/87
  [VINP_RRRawWhlSpeedV_flg] -> bus_creator/88
  [VINP_RRWhlRotDir_enum] -> bus_creator/89
  [VINP_RearAxlTrqReqDrv_Nm] -> bus_creator/90
  [VINP_RedWnlmpSta_flg] -> bus_creator/91
  [VINP_RrPTCSActive_flg] -> bus_creator/92
  [VINP_TCSActive_flg] -> bus_creator/93
  [VINP_TCSFailed_flg] -> bus_creator/94
  [VINP_VehSpeed_kph] -> bus_creator/95
  [VINP_ESC5CSErr_flg] -> bus_creator/96
  [VINP_ESC5RCErr_flg] -> bus_creator/97
  [VINP_ACCAvail_flg] -> bus_creator/98
  [VINP_AEBAvail_flg] -> bus_creator/99
  [VINP_ActBrkLampSta_flg] -> bus_creator/100
  [VINP_BrkDiscTempSta_flg] -> bus_creator/101
  [VINP_BrkPedalPos_pct] -> bus_creator/102
  [VINP_BrkPedalPosSta_flg] -> bus_creator/103
  [VINP_BrkSwSta_flg] -> bus_creator/104
  [VINP_BrkSwV_flg] -> bus_creator/105
  [VINP_ESC5CS_enum] -> bus_creator/106
  [VINP_ESC5RC_enum] -> bus_creator/107
  [VINP_ESCADASSta_enum] -> bus_creator/108
  [VINP_ESCAPSSta_enum] -> bus_creator/109
  [VINP_ESCStandstill_flg] -> bus_creator/110
  [VINP_FrRBCActive_flg] -> bus_creator/111
  [VINP_FrntAxlTrqReqBrk_Nm] -> bus_creator/112
  [VINP_LatAccel_Gps] -> bus_creator/113
  [VINP_LatAccelV_flg] -> bus_creator/114
  [VINP_LongAccel_Gps] -> bus_creator/115
  [VINP_LongAccelV_flg] -> bus_creator/116
  [VINP_MCPressure_bar] -> bus_creator/117
  [VINP_MCPressureV_flg] -> bus_creator/118
  [VINP_MeterIndVehSpeed_kph] -> bus_creator/119
  [VINP_RDCActive_enum] -> bus_creator/120
  [VINP_RearAxlTrqReqBrk_Nm] -> bus_creator/121
  [VINP_RrRBCActive_flg] -> bus_creator/122
  [VINP_YawRate_degps] -> bus_creator/123
  [VINP_YawRateV_flg] -> bus_creator/124
  [VINP_LowBrakeFluidSta_flg] -> bus_creator/125
  [VINP_eBSTAmberWnlmpSta_flg] -> bus_creator/126
  [VINP_eBSTBeepReq_flg] -> bus_creator/127
  [VINP_eBSTRedWnlmpSta_flg] -> bus_creator/128

== system inp/INP/CAN2/CommunicationCheck ==
  BHAL_outputs : Inport
  CANMsgInvalidHMI1 : FVT_lib/inp/CAN_Msg_Validity_Process_template  SystemSampleTime=-1  VariantActivationTime=update diagram  Latency=0  AutoFrameSizeCalculation=off
      link override ovrdflg: Value=KINP_CANMsgInvalidHMI1_flg_ovrdflg
      link override ovrdval: Value=KINP_CANMsgInvalidHMI1_flg_ovrdval
  CANMsgInvalidIVI1 : FVT_lib/inp/CAN_Msg_Validity_Process_template  SystemSampleTime=-1  VariantActivationTime=update diagram  Latency=0  AutoFrameSizeCalculation=off
      link override ovrdflg: Value=KINP_CANMsgInvalidIVI1_flg_ovrdflg
      link override ovrdval: Value=KINP_CANMsgInvalidIVI1_flg_ovrdval
  CANMsgInvalidIVI2 : FVT_lib/inp/CAN_Msg_Validity_Process_template  SystemSampleTime=-1  VariantActivationTime=update diagram  Latency=0  AutoFrameSizeCalculation=off
      link override ovrdflg: Value=KINP_CANMsgInvalidIVI2_flg_ovrdflg
      link override ovrdval: Value=KINP_CANMsgInvalidIVI2_flg_ovrdval
  CANMsgInvalidIVI3 : FVT_lib/inp/CAN_Msg_Validity_Process_template  SystemSampleTime=-1  VariantActivationTime=update diagram  Latency=0  AutoFrameSizeCalculation=off
      link override ovrdflg: Value=KINP_CANMsgInvalidIVI3_flg_ovrdflg
      link override ovrdval: Value=KINP_CANMsgInvalidIVI3_flg_ovrdval
  CANMsgInvalidMETER1 : FVT_lib/inp/CAN_Msg_Validity_Process_template  SystemSampleTime=-1  VariantActivationTime=update diagram  Latency=0  AutoFrameSizeCalculation=off
      link override ovrdflg: Value=KINP_CANMsgInvalidMETER1_flg_ovrdflg
      link override ovrdval: Value=KINP_CANMsgInvalidMETER1_flg_ovrdval
  bus_creator : BusCreator  Inputs=5
  bus_selector : BusSelector  OutputSignals=VHAL_CANMsgInvalidHMI1_flg,VHAL_CANMsgInvalidIVI1_flg,VHAL_CANMsgInvalidIVI2_flg,VHAL_CANMsgInvalidIVI3_flg,VHAL_CANMsgInvalidMETER1_flg
  not{1..5} (5 alike) : Logic  Operator=NOT  AllPortsSameDT=off  OutDataTypeStr=boolean
  inp_CanValid_bus : Outport
  wires:
  BHAL_outputs/1 -> [BHAL_outputs]
  bus_selector/1 -> CANMsgInvalidHMI1/1  "<VHAL_CANMsgInvalidHMI1_flg>"
  CANMsgInvalidHMI1/1 -> not1/1
  not1/1 -> bus_creator/1  "VINP_CANMsgValidHMI1_flg"
  bus_selector/2 -> CANMsgInvalidIVI1/1  "<VHAL_CANMsgInvalidIVI1_flg>"
  CANMsgInvalidIVI1/1 -> not2/1
  not2/1 -> bus_creator/2  "VINP_CANMsgValidIVI1_flg"
  bus_selector/3 -> CANMsgInvalidIVI2/1  "<VHAL_CANMsgInvalidIVI2_flg>"
  CANMsgInvalidIVI2/1 -> not3/1
  not3/1 -> bus_creator/3  "VINP_CANMsgValidIVI2_flg"
  bus_selector/4 -> CANMsgInvalidIVI3/1  "<VHAL_CANMsgInvalidIVI3_flg>"
  CANMsgInvalidIVI3/1 -> not4/1
  not4/1 -> bus_creator/4  "VINP_CANMsgValidIVI3_flg"
  bus_selector/5 -> CANMsgInvalidMETER1/1  "<VHAL_CANMsgInvalidMETER1_flg>"
  CANMsgInvalidMETER1/1 -> not5/1
  not5/1 -> bus_creator/5  "VINP_CANMsgValidMETER1_flg"
  [BHAL_outputs] -> bus_selector/1
  bus_creator/1 -> inp_CanValid_bus/1
